simulink model "temp"  (R2025b)
settings: Solver=VariableStepAuto  StartTime=0.0  StopTime=simlength  RelTol=1e-3
values from neighbouring files (symbols this model uses):
  dT_base = 0.1e-3    (= 0.0001)    [init_dtg.m]    (also in init_dtmp_analysis.m = 0.0004)
  N = 10    [init_dtg.m]    (also in init_dtmp_analysis.m = 40)
  Ton_base = 1e-6    (= 1e-06)    [init_dtg.m]    (also in init_dtmp_analysis.m = 3.33e-07)
  vin_cmd = 15    [init_dtg.m]    (also in init_dtmp_analysis.m)
settings Model: Creator=dbagn  LastModifiedBy=dbagn

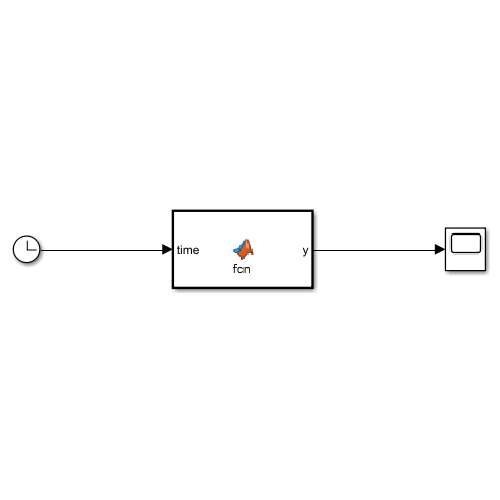
[thumbnail: Simulink's stored preview of the top-level diagram]
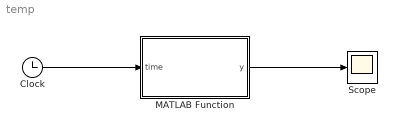
== system temp ==
  Clock : Clock
  MATLAB Function : MATLAB Function  TreatAsAtomicUnit=on
  Scope : Scope
      settings: SampleTime=tc  ActiveDisplayYMinimum=-1.8749999999999996  ActiveDisplayYMaximum=16.875
  wires:
  Clock/1 -> MATLAB Function/1(time)
  MATLAB Function/1(y) -> Scope/1

== matlab function temp/MATLAB Function ==
  data: time input; y output; Ton_base parameter; dT_base parameter; vin_cmd parameter; N parameter
function y = fcn(time, Ton_base, dT_base, vin_cmd, N)
    y = 0;
    
    for n = 1:N
        if (time >= n*dT_base && time <= (n*dT_base + n*Ton_base))
            y = vin_cmd;
            break;
        end
    end
end
